simulink model "pll_fsk"  (Simulink 6.0)
settings: Solver=ode45  StartTime=0.0  StopTime=1.5  RelTol=1e-3
libraries: commsynccomp2 x2
settings Model: LastModifiedBy=estel

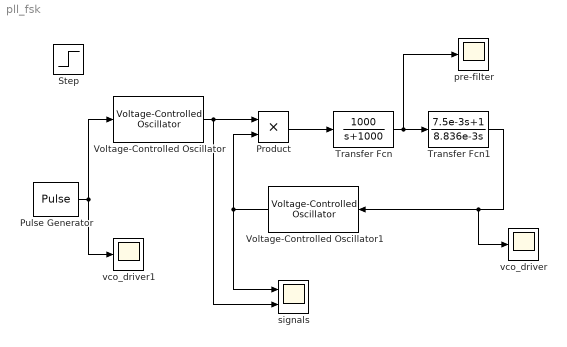
== system pll_fsk ==
  Product : Product  RndMeth=Zero
  Pulse Generator : DiscretePulseGenerator  PulseType=Time based  Period=0.5  PulseWidth=50  SampleTime=3e-6
  Step : Step  Time=10e-3  SampleTime=3e-6
  Transfer Fcn : TransferFcn  Numerator=[1000]  Denominator=[1 1000]
  Transfer Fcn1 : TransferFcn  Numerator=[7.5e-3 1]  Denominator=[8.836e-3 0]
  Voltage-Controlled Oscillator : commsynccomp2/Voltage-Controlled Oscillator  Ac=1  Fc=5000  Kc=100  Ph=0
  Voltage-Controlled Oscillator1 : commsynccomp2/Voltage-Controlled Oscillator  Orientation=left  Ac=1  Fc=5000  Kc=70  Ph=0
  pre-filter : Scope
      settings: YMin=-1  YMax=2  SaveName=ScopeData2  SampleInput=on
  signals : Scope  NumInputPorts=2
      settings: TimeRange=0.000980392156865  YMin=-2~-2  YMax=2~2  SampleInput=on
  vco_driver : Scope
      settings: YMin=-1  YMax=2  SampleInput=on
  vco_driver1 : Scope
      settings: YMin=-1  YMax=2  SaveName=ScopeData3  SampleInput=on
  wires:
  Voltage-Controlled Oscillator/1 -> Product/1, signals/2
  Voltage-Controlled Oscillator1/1 -> Product/2, signals/1
  Product/1 -> Transfer Fcn/1
  Transfer Fcn/1 -> Transfer Fcn1/1, pre-filter/1
  Transfer Fcn1/1 -> Voltage-Controlled Oscillator1/1, vco_driver/1
  Pulse Generator/1 -> Voltage-Controlled Oscillator/1, vco_driver1/1
